simulink model "chap6_3sim"  (Simulink 8.1)
settings: Solver=ode45  StartTime=0.0  StopTime=30  RelTol=1e-3
settings Model: Creator=Administrator  LastModifiedBy=liujk
settings DataIOCC: SignalLoggingName=sigsOut
settings OptimizationCC: InitFltsAndDblsToZero=on
settings DebuggingCC: SaveWithParameterizedLinksMsg=none  SignalResolutionControl=TryResolveAllWithWarning  SolverPrmCheckMsg=none  MultiTaskDSMMsg=warning  MultiTaskCondExecSysMsg=none  StrictBusMsg=None
settings HardwareCC: TargetUnknown=on
settings RTWCC: IncludeERTFirstTime=on
settings GRTTargetCC: TargetFcnLib=ansi_tfl_tmw.mat

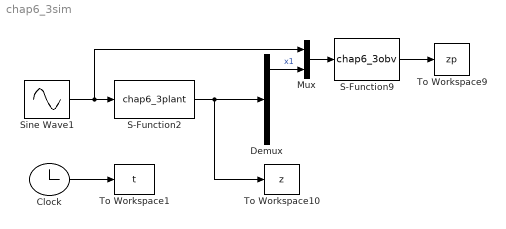
== system chap6_3sim ==
  Clock : Clock
  Demux : Demux
  Mux : Mux  Inputs=2
  S-Function2 : S-Function  FunctionName=chap6_3plant  EnableBusSupport=off
  S-Function9 : S-Function  FunctionName=chap6_3obv  EnableBusSupport=off
  Sine Wave1 : Sin  SampleTime=0
  To Workspace1 : ToWorkspace  VariableName=t  SampleTime=-1
  To Workspace10 : ToWorkspace  VariableName=z  SampleTime=-1
  To Workspace9 : ToWorkspace  VariableName=zp  SampleTime=-1
  wires:
  Clock/1 -> To Workspace1/1
  Sine Wave1/1 -> S-Function2/1, Mux/1
  S-Function2/1 -> To Workspace10/1, Demux/1
  S-Function9/1 -> To Workspace9/1
  Mux/1 -> S-Function9/1
  Demux/1 -> Mux/2  "x1"
